simulink model "solar_collector"  (R2017a)
settings: Solver=FixedStepAuto  StartTime=0.0  StopTime=50000  RelTol=1e-3
values from neighbouring files (symbols this model uses):
  a1 = Ac*eta/C_c    (= 0.000575964912281)    [Linearized_model.m]    (also in Linearized_model_v1.m; Maple_linearization.m = 0.000380952380952; solar_collector_init.m = 7.33988724098e-05)
  a2 = -U_L1*Ac/2/C_c    (= -0.00145487240829)    [Linearized_model.m]    (also in Linearized_model_v1.m = -0.00290974481659; Maple_linearization.m = 0.00111111111111; solar_collector_init.m = -0.000214080044529)
  a3 = -U_L2*Ac/C_c    (= -7.48006379585e-06)    [Linearized_model.m]    (also in Linearized_model_v1.m; Maple_linearization.m = -0.00222222222222; solar_collector_init.m = 0.000428160089057)
  a4 = V_c^-1    (= 333.333333333)    [Linearized_model.m]    (also in Linearized_model_v1.m; Maple_linearization.m = 666.666666667; solar_collector_init.m = 133.333333333)
  a5 = -a4    (= -333.333333333)    [Linearized_model.m]    (also in Linearized_model_v1.m; Maple_linearization.m = -666.666666667; solar_collector_init.m = -133.333333333)
settings Model: Creator=info  LastModifiedBy=info

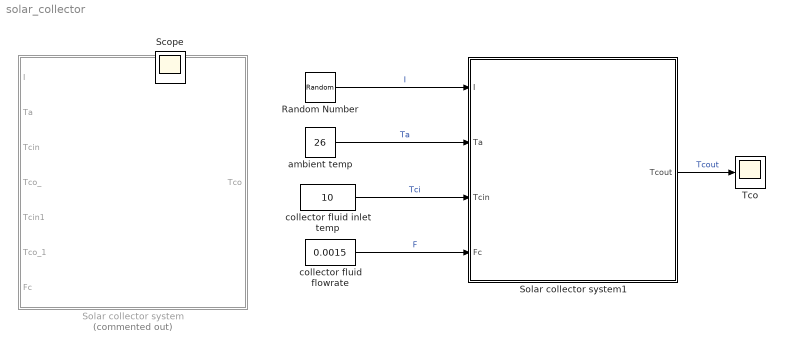
== system solar_collector ==
  Random Number : RandomNumber  Mean=12000  SampleTime=0.1
  Solar collector system : Subsystem  Commented=on
      mask Display: image('collector_image.jpg');
  Solar collector system1 : Subsystem
      mask Display: image('collector_image.jpg');
  Tco : Scope
  ambient temp : Constant  Value=26
  collector fluid flowrate : Constant  Value=0.0015
  collector fluid inlet temp : Constant  Value=10
  Scope : Scope
  wires:
  Random Number/1 -> Solar collector system1/1(I)  "I"
  ambient temp/1 -> Solar collector system1/2(Ta)  "Ta"
  collector fluid inlet temp/1 -> Solar collector system1/3(Tcin)  "Tci"
  collector fluid flowrate/1 -> Solar collector system1/4(Fc)  "F"
  Solar collector system1/1(Tcout) -> Tco/1  "Tcout"

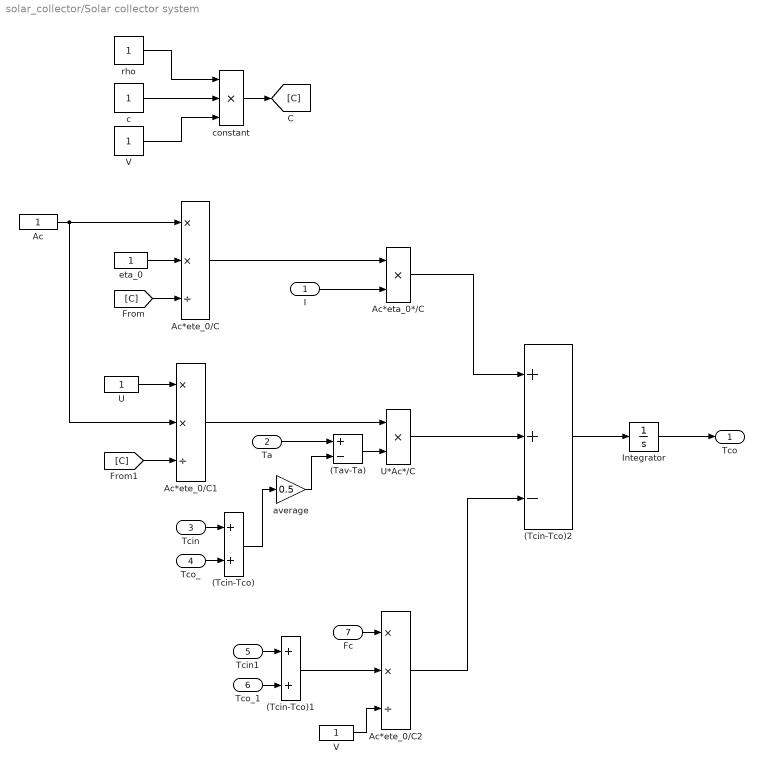
== system solar_collector/Solar collector system ==
  I : Inport
  Ta : Inport  Port=2
  Tcin : Inport  Port=3
  Tco_ : Inport  Port=4
  Tcin1 : Inport  Port=5
  Tco_1 : Inport  Port=6
  Fc : Inport  Port=7
  (Tav-Ta) : Sum  Inputs=+-
  (Tcin-Tco) : Sum
  (Tcin-Tco)1 : Sum
  (Tcin-Tco)2 : Sum  Inputs=++-
  Ac : Constant
  Ac*eta_0*/C : Product  Inputs=**
  Ac*ete_0/C : Product  Inputs=**/
  Ac*ete_0/C1 : Product  Inputs=**/
  Ac*ete_0/C2 : Product  Inputs=**/
  Integrator : Integrator
  U : Constant
  U*Ac*/C : Product  Inputs=**
  V : Constant
  "V   " : Constant
  average : Gain  Gain=0.5
  c : Constant
  "constant " : Product  Inputs=***
  "eta_0 " : Constant
  rho : Constant
  Tco : Outport
  wires:
  rho/1 -> "constant "/1
  c/1 -> "constant "/2
  V/1 -> "constant "/3
  "constant "/1 -> [C]
  Ac/1 -> Ac*ete_0/C1/2, Ac*ete_0/C/1
  "eta_0 "/1 -> Ac*ete_0/C/2
  [C] -> Ac*ete_0/C/3
  Ac*ete_0/C/1 -> Ac*eta_0*/C/1
  I/1 -> Ac*eta_0*/C/2
  U/1 -> Ac*ete_0/C1/1
  [C] -> Ac*ete_0/C1/3
  Ac*ete_0/C1/1 -> U*Ac*/C/1
  (Tav-Ta)/1 -> U*Ac*/C/2
  Ta/1 -> (Tav-Ta)/1
  (Tcin-Tco)/1 -> average/1
  average/1 -> (Tav-Ta)/2
  Tcin/1 -> (Tcin-Tco)/1
  Tco_/1 -> (Tcin-Tco)/2
  Tcin1/1 -> (Tcin-Tco)1/1
  Tco_1/1 -> (Tcin-Tco)1/2
  (Tcin-Tco)1/1 -> Ac*ete_0/C2/2
  "V   "/1 -> Ac*ete_0/C2/3
  Fc/1 -> Ac*ete_0/C2/1
  (Tcin-Tco)2/1 -> Integrator/1
  Integrator/1 -> Tco/1
  Ac*eta_0*/C/1 -> (Tcin-Tco)2/1
  U*Ac*/C/1 -> (Tcin-Tco)2/2
  Ac*ete_0/C2/1 -> (Tcin-Tco)2/3

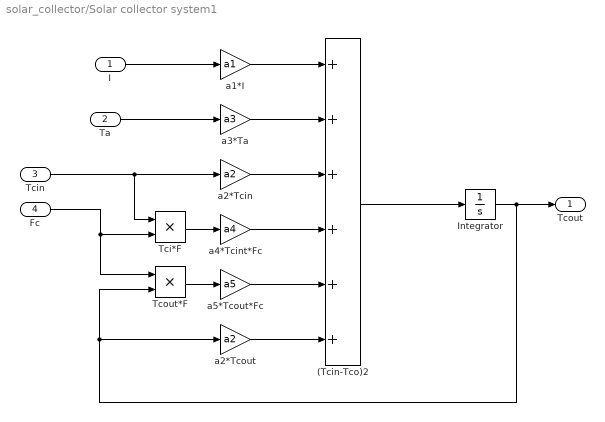
== system solar_collector/Solar collector system1 ==
  I : Inport
  Ta : Inport  Port=2
  Tcin : Inport  Port=3
  Fc : Inport  Port=4
  (Tcin-Tco)2 : Sum  Inputs=++++++
  Integrator : Integrator  InitialCondition=10
  Tci*F : Product  Inputs=**
  Tcout*F : Product  Inputs=**
  a1*I : Gain  Gain=a1
  a2*Tcin : Gain  Gain=a2
  "a2*Tcout " : Gain  Gain=a2
  a3*Ta : Gain  Gain=a3
  a4*Tcint*Fc : Gain  Gain=a4
  "a5*Tcout*Fc " : Gain  Gain=a5
  Tcout : Outport
  wires:
  I/1 -> a1*I/1
  Integrator/1 -> "a2*Tcout "/1, Tcout*F/2, Tcout/1
  (Tcin-Tco)2/1 -> Integrator/1
  Fc/1 -> Tcout*F/1, Tci*F/2
  a1*I/1 -> (Tcin-Tco)2/1
  Ta/1 -> a3*Ta/1
  Tcin/1 -> Tci*F/1, a2*Tcin/1
  a3*Ta/1 -> (Tcin-Tco)2/2
  a2*Tcin/1 -> (Tcin-Tco)2/3
  "a5*Tcout*Fc "/1 -> (Tcin-Tco)2/5
  Tci*F/1 -> a4*Tcint*Fc/1
  a4*Tcint*Fc/1 -> (Tcin-Tco)2/4
  Tcout*F/1 -> "a5*Tcout*Fc "/1
  "a2*Tcout "/1 -> (Tcin-Tco)2/6
